simulink model "L4_eu1"  (Simulink 7.9)
settings: Solver=ode45  StartTime=0.0  StopTime=10.0  RelTol=1e-3
values from neighbouring files (symbols this model uses):
  A1 = [-(Rg+Ron+Rp)/(Lm*(n^2))  -R/((R+Rc)*n*Lm); R/((R+Rc)*n*C)  -1/((R+Rc)*C)]    [ESR.m]    (also in b.m; c.m; d.m = [-(Ron+Rg+Rp)/(n^2*Lm) -R/(n*Lm*(R+Rc)); R/((R+Rc)*n*C) -1/(; g2.m = [-(Ron+Rg+Rp)/(n^2*Lm) -R/(n*Lm*(R+Rc)); R/((R+Rc)*n*C) -1/()
  A2 = [-Rp/(Lm*((n+1)^2))  -R/((n+1)*(R+Rc)*Lm); R/((n+1)*(R+Rc)*C)  -1/((R+Rc)*C)]    [ESR.m]    (also in b.m; c.m; d.m = [-Rp/((n+1)^2*Lm) -R/((n+1)*Lm*(R+Rc)); R/((n+1)*(R+Rc)*C) -; g2.m = [-Rp/((n+1)^2*Lm) -R/((n+1)*Lm*(R+Rc)); R/((n+1)*(R+Rc)*C) -)
  B1 = [1/(n*Lm)  -1/(n*Lm)  0  0 0; 0  0  0  0 0]    [ESR.m]    (also in b.m; c.m; d.m = [1/(n*Lm) -1/(n*Lm) 0 0; 0 0 0 0]; g2.m = [1/(n*Lm) -1/(n*Lm) 0 0; 0 0 0 0])
  B2 = [0  0  -1/((n+1)*Lm)  -1/(Lm*(n+1)) 0; 0  0  0  0 0]    [ESR.m]    (also in b.m; c.m; d.m = [0 0 -1/((n+1)*Lm) -1/((n+1)*Lm); 0 0 0 0]; g2.m = [0 0 -1/((n+1)*Lm) -1/((n+1)*Lm); 0 0 0 0])
  C1 = [1 0; Rp/n R/(R+Rc); 1/n 0]    [d.m]
  C2 = [1 0; Rp/(n+1) R/(R+Rc); 0 0]    [d.m]
  D1 = [0 0 0 0; 0 0 0 0; 0 0 0 0]    [d.m]
  D2 = [0 0 0 0; 0 0 0 0; 0 0 0 0]    [d.m]
settings Model: Creator=Student  LastModifiedBy=ghita
settings OptimizationCC: InitFltsAndDblsToZero=on
settings DebuggingCC: FcnCallInpInsideContextMsg=Use local settings  StrictBusMsg=Warning
settings GRTTargetCC: CombineOutputUpdateFcns=off  GRTInterface=on

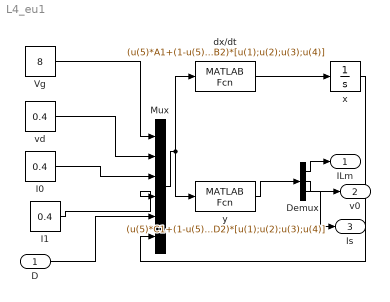
== system L4_eu1 ==
  D : Inport
  Demux : Demux  Outputs=3
  I0 : Constant  Value=0.4
  I1 : Constant  Value=0.4
  Mux : Mux  Inputs=6
  Vg : Constant  Value=8
  dx/dt : MATLABFcn  MATLABFcn=(u(5)*A1+(1-u(5))*A2)*[u(6);u(7)]+(u(5)*B1+(1-u(5))*B2)*[u(1);u(2);u(3);u(4)]  OutputDimensions=2
  vd : Constant  Value=0.4
  x : Integrator
  y : MATLABFcn  MATLABFcn=(u(5)*C1+(1-u(5))*C2)*[u(6);u(7)]+(u(5)*D1+(1-u(5))*D2)*[u(1);u(2);u(3);u(4)]  OutputDimensions=3  Output1D=off
  ILm : Outport
  v0 : Outport  Port=2
  Is : Outport  Port=3
  wires:
  dx/dt/1 -> x/1
  Vg/1 -> Mux/1
  Mux/1 -> dx/dt/1, y/1
  y/1 -> Demux/1
  Demux/1 -> ILm/1
  Demux/2 -> v0/1
  vd/1 -> Mux/2
  I0/1 -> Mux/3
  I1/1 -> Mux/4
  D/1 -> Mux/5
  x/1 -> Mux/6
  Demux/3 -> Is/1
